simulink model "MotorDC"  (R2022a)
settings: Solver=VariableStepAuto  StartTime=0.0  StopTime=10.0  RelTol=1e-3
settings Model: Creator=andre  LastModifiedBy=andre

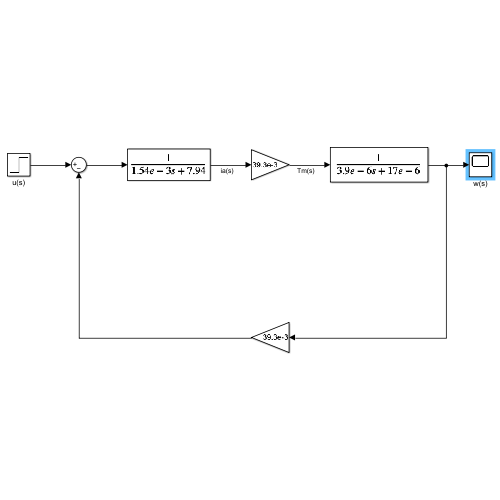
[thumbnail: Simulink's stored preview of the top-level diagram]
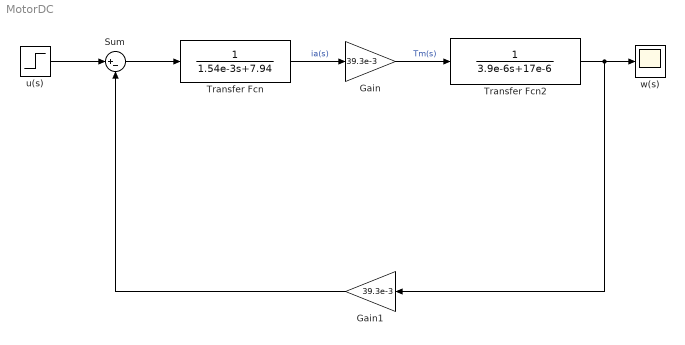
== system MotorDC ==
  Gain : Gain  Gain=39.3e-3
  Gain1 : Gain  Gain=39.3e-3
  Sum : Sum  Inputs=|+-
  Transfer Fcn : TransferFcn  Denominator=[1.54e-3 7.94]
  Transfer Fcn2 : TransferFcn  Denominator=[3.9e-6 17e-6]
  u(s) : Step  SampleTime=0
  w(s) : Scope
  wires:
  Transfer Fcn/1 -> Gain/1  "ia(s)"
  u(s)/1 -> Sum/1
  Sum/1 -> Transfer Fcn/1
  Gain/1 -> Transfer Fcn2/1  "Tm(s)"
  Transfer Fcn2/1 -> w(s)/1, Gain1/1
  Gain1/1 -> Sum/2
